simulink model "WorkshopB_1"  (R2016a)
settings: Solver=ode45  SolverMode=SingleTasking  StartTime=0.0  StopTime=5  RelTol=1e-3
values from neighbouring files (symbols this model uses):
  dm = dm*eps_dm    (= 1.3528e-05)    [param.m]
  Dpos = double(D)    [param.m]
  Fc = 0.0013    [param.m]
  Ipos = double(I)    [param.m]
  Jeq = eps_Jeq*Jeq    (= 2.20476e-05)    [param.m]
  Kemf = 1/(137*2*pi/60)    (= 0.0697028947848)    [param.m]
  Km = 69.7E-3    (= 0.0697)    [param.m]
  n = 1    [param.m]
  Npos = double(N)    [param.m]
  Ppos = double(P)    [param.m]
  R = s*s + s*N    [PID_calc.m]    (also in param.m = 112)
  Ts = 5e-3    (= 0.005)    [param.m]
undefined symbols (not defined in the file or in its folder): DiscIntNeverNeededParam, sigbuilder_block
settings Model: Creator=sofianh  LastModifiedBy=diegogm
settings DataIOCC: LimitDataPoints=on  SaveFormat=Array
settings OptimizationCC: BlockReduction=off  BooleanDataType=off
settings DebuggingCC: SaveWithParameterizedLinksMsg=none  UnderspecifiedInitializationDetection=Classic  MergeDetectMultiDrivingBlocksExec=none  SignalResolutionControl=TryResolveAllWithWarning
settings HardwareCC: ProdBitPerPointer=32  ProdLargestAtomicFloat=None  ProdIntDivRoundTo=Undefined  ProdEndianess=Unspecified  ProdWordSize=32  ProdHWDeviceType=32-bit Generic  TargetUnknown=on
settings ModelReferenceCC: PropagateSignalLabelsOutOfModel=off
settings ConfigComp: CovModelRefEnable=Off  CovSFcnEnable=off

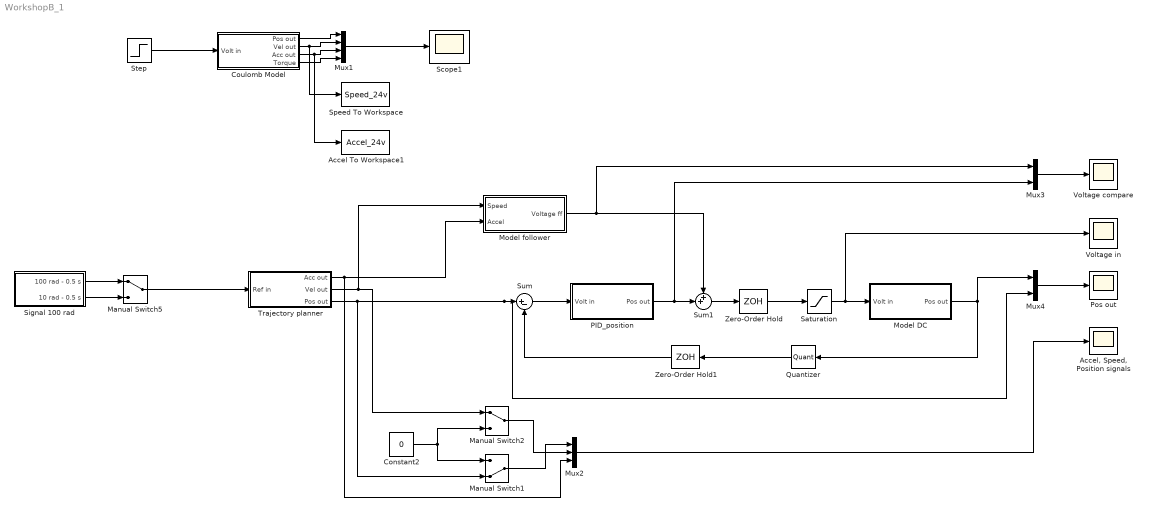
== system WorkshopB_1 ==
  Accel To Workspace1 : ToWorkspace  VariableName=Accel_24v  SaveFormat=Timeseries  SampleTime=-1
  "Accel, Speed, Position signals" : Scope
  Constant2 : Constant  Value=0
  Coulomb Model : Subsystem
  Manual Switch1 : ManualSwitch  CurrentSetting=0
  Manual Switch2 : ManualSwitch
  Manual Switch5 : ManualSwitch
  "Model DC " : Subsystem
  Model follower : Subsystem
  Mux1 : Mux
  Mux2 : Mux  Inputs=3
  Mux3 : Mux  Inputs=2
  Mux4 : Mux  Inputs=2
  PID_position : Subsystem
  Pos out : Scope
  Quantizer : Quantizer  QuantizationInterval=Pulses  SampleTime=Ts
  Saturation : Saturate  UpperLimit=24  LowerLimit=-24
  Scope1 : Scope
  Signal 100 rad : Subsystem  Tag=STV Subsys  LoadFcn=sigbuilder_block('load',[437.6 199.2 550.4 400 ]);  StartFcn=sigbuilder_block('start');  StopFcn=sigbuilder_block('stop');  ClipboardFcn=sigbuilder_block('clipboard');  mask(Sigbuilder block){}
      mask help: Simulink:masks:SigbuilderBlock_MD
      mask init:
      | if ~strcmp(get_param(bdroot(gcbh),'SimulationStatus'),'stopped') tuvar = sigbuilder_block('maskInit'); end
      settings: CopyFcn=sigbuilder_block('copy');  DeleteFcn=sigbuilder_block('delete');  ModelCloseFcn=sigbuilder_block('modelClose');  PreSaveFcn=sigbuilder_block('preSave');  PauseFcn=sigbuilder_block('pause');  ContinueFcn=sigbuilder_block('continue');  NameChangeFcn=sigbuilder_block('namechange');  OpenFcn=sigbuilder_block('open',[437.6 199.2 550.4 400 ]);  CloseFcn=sigbuilder_block('close');
      mask Display: plot(0, 0, 100, 100,[2, 2, 32, 32, 2], [68, 8, 8, 68, 68],[32, 2], [38, 38], [32, 19, 2],[53, 60, 44], [32, 17, 17, 2],[16, 16, 31, 31]);txt = getActiveGroup(gcbh);text(2, 100, txt,'verticalAlignment', 'top');
  Speed To Workspace : ToWorkspace  VariableName=Speed_24v  SaveFormat=Timeseries  SampleTime=-1
  Step : Step  Time=0  After=24  SampleTime=0
  Sum : Sum  Inputs=|+-
  Sum1 : Sum  Inputs=++|
  Trajectory planner : Subsystem
  Voltage compare : Scope
  Voltage in : Scope
  Zero-Order Hold : ZeroOrderHold  SampleTime=Ts
  Zero-Order Hold1 : ZeroOrderHold  SampleTime=Ts
  wires:
  Mux1/1 -> Scope1/1
  Coulomb Model/1(Pos out) -> Mux1/1
  Step/1 -> Coulomb Model/1(Volt in)
  Coulomb Model/2(Vel out) -> Speed To Workspace/1, Mux1/2
  Coulomb Model/3(Acc out) -> Accel To Workspace1/1, Mux1/3
  Coulomb Model/4(Torque) -> Mux1/4
  Mux2/1 -> "Accel, Speed, Position signals"/1
  Manual Switch1/1 -> Mux2/1
  Manual Switch2/1 -> Mux2/2
  Constant2/1 -> Manual Switch2/2, Manual Switch1/1
  Sum/1 -> PID_position/1(Volt in)
  "Model DC "/1(Pos out) -> Quantizer/1, Mux4/1
  PID_position/1(Pos out) -> Mux3/2, Sum1/2
  Mux3/1 -> Voltage compare/1
  Model follower/1(Voltage ff) -> Sum1/1, Mux3/1
  Mux4/1 -> Pos out/1
  Trajectory planner/1("Acc out ") -> Model follower/2(Accel), Mux2/3
  Trajectory planner/2(Vel out) -> Manual Switch2/1, Model follower/1(Speed)
  Trajectory planner/3("Pos out ") -> Mux4/2, Sum/1, Manual Switch1/2
  Sum1/1 -> Zero-Order Hold/1
  Quantizer/1 -> Zero-Order Hold1/1
  Zero-Order Hold1/1 -> Sum/2
  Manual Switch5/1 -> Trajectory planner/1(Ref in)
  Signal 100 rad/1(100 rad - 0.5 s) -> Manual Switch5/1
  Signal 100 rad/2(10 rad - 0.5 s) -> Manual Switch5/2
  Zero-Order Hold/1 -> Saturation/1
  Saturation/1 -> Voltage in/1, "Model DC "/1("Volt in ")

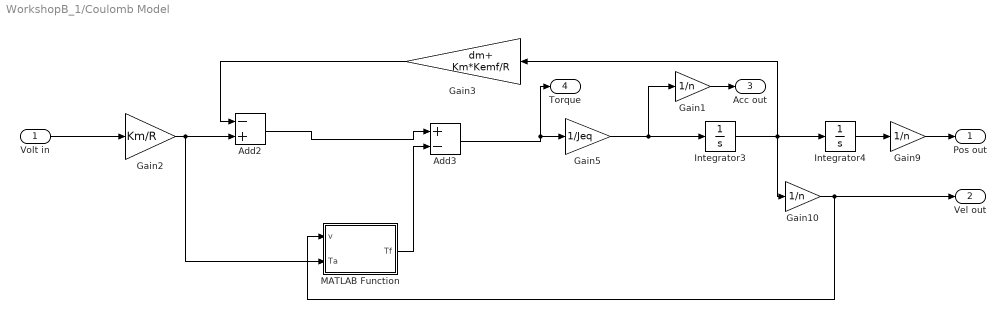
== system WorkshopB_1/Coulomb Model ==
  Volt in : Inport
  Add2 : Sum  Inputs=-+
  Add3 : Sum  Inputs=+-
  Gain1 : Gain  Gain=1/n
  Gain10 : Gain  Gain=1/n
  Gain2 : Gain  Gain=Km/R
  Gain3 : Gain  Gain=dm+ Km*Kemf/R
  Gain5 : Gain  Gain=1/Jeq
  Gain9 : Gain  Gain=1/n
  Integrator3 : Integrator
  Integrator4 : Integrator
  MATLAB Function : MATLAB Function  TreatAsAtomicUnit=on
  Pos out : Outport
  Vel out : Outport  Port=2
  Acc out : Outport  Port=3
  Torque : Outport  Port=4
  wires:
  Gain2/1 -> MATLAB Function/2(Ta), Add2/2
  Integrator3/1 -> Integrator4/1, Gain10/1, Gain3/1
  Gain3/1 -> Add2/1
  Gain5/1 -> Integrator3/1, Gain1/1
  Integrator4/1 -> Gain9/1
  Gain10/1 -> Vel out/1, MATLAB Function/1(v)
  Volt in/1 -> Gain2/1
  Add3/1 -> Torque/1, Gain5/1
  Add2/1 -> Add3/1
  MATLAB Function/1(Tf) -> Add3/2
  Gain9/1 -> Pos out/1
  Gain1/1 -> Acc out/1

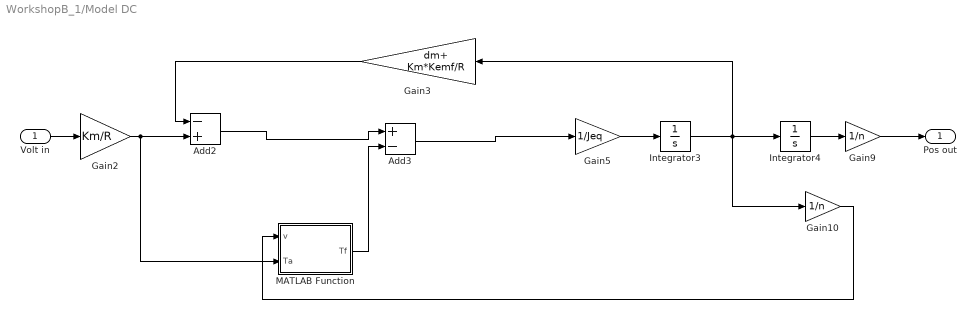
== system WorkshopB_1/Model DC  ==
  "Volt in " : Inport
  Add2 : Sum  Inputs=-+
  Add3 : Sum  Inputs=+-
  Gain10 : Gain  Gain=1/n
  Gain2 : Gain  Gain=Km/R
  Gain3 : Gain  Gain=dm+ Km*Kemf/R
  Gain5 : Gain  Gain=1/Jeq
  Gain9 : Gain  Gain=1/n
  Integrator3 : Integrator
  Integrator4 : Integrator
  MATLAB Function : MATLAB Function  TreatAsAtomicUnit=on
  Pos out : Outport
  wires:
  Gain2/1 -> MATLAB Function/2(Ta), Add2/2
  Integrator3/1 -> Integrator4/1, Gain10/1, Gain3/1
  Gain3/1 -> Add2/1
  Gain5/1 -> Integrator3/1
  Integrator4/1 -> Gain9/1
  Gain10/1 -> MATLAB Function/1(v)
  Add3/1 -> Gain5/1
  Add2/1 -> Add3/1
  MATLAB Function/1(Tf) -> Add3/2
  "Volt in "/1 -> Gain2/1
  Gain9/1 -> Pos out/1

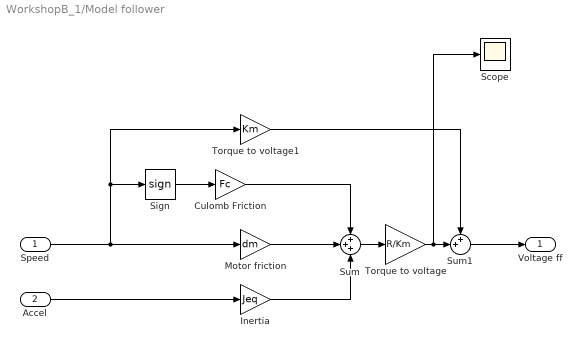
== system WorkshopB_1/Model follower ==
  Speed : Inport
  Accel : Inport  Port=2
  Culomb Friction : Gain  Gain=Fc
  "Inertia " : Gain  Gain=Jeq
  Motor friction : Gain  Gain=dm
  Scope : Scope
  Sign : Signum
  Sum : Sum  Inputs=+++
  Sum1 : Sum  Inputs=++|
  Torque to voltage : Gain  Gain=R/Km
  Torque to voltage1 : Gain  Gain=Km
  Voltage ff : Outport
  wires:
  Accel/1 -> "Inertia "/1
  Speed/1 -> Torque to voltage1/1, Sign/1, Motor friction/1
  "Inertia "/1 -> Sum/3
  Motor friction/1 -> Sum/2
  Sum/1 -> Torque to voltage/1
  Torque to voltage1/1 -> Sum1/1
  Torque to voltage/1 -> Scope/1, Sum1/2
  Sum1/1 -> Voltage ff/1
  Sign/1 -> Culomb Friction/1
  Culomb Friction/1 -> Sum/1

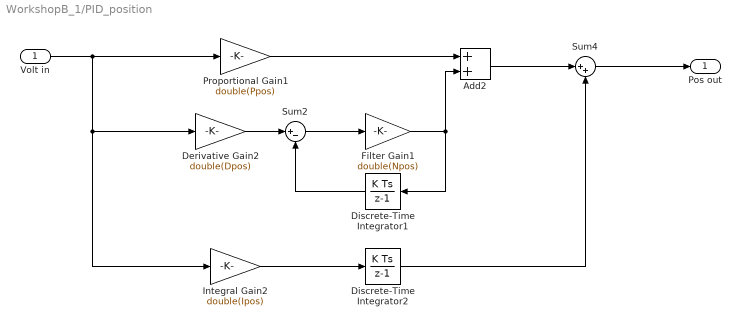
== system WorkshopB_1/PID_position ==
  Volt in : Inport
  Add2 : Sum
  Derivative Gain2 : Gain  Gain=double(Dpos)
  Discrete-Time Integrator1 : DiscreteIntegrator  InitialConditionSetting=State (most efficient)  SampleTime=Ts  ICPrevOutput=DiscIntNeverNeededParam  ICPrevScaledInput=DiscIntNeverNeededParam
  Discrete-Time Integrator2 : DiscreteIntegrator  InitialConditionSetting=State (most efficient)  SampleTime=Ts  ICPrevOutput=DiscIntNeverNeededParam  ICPrevScaledInput=DiscIntNeverNeededParam
  Filter Gain1 : Gain  Gain=double(Npos)
  Integral Gain2 : Gain  Gain=double(Ipos)
  Proportional Gain1 : Gain  Gain=double(Ppos)
  Sum2 : Sum  Inputs=|+-
  Sum4 : Sum  Inputs=|++
  Pos out : Outport
  wires:
  Discrete-Time Integrator2/1 -> Sum4/2
  Add2/1 -> Sum4/1
  Volt in/1 -> Integral Gain2/1, Derivative Gain2/1, Proportional Gain1/1
  Discrete-Time Integrator1/1 -> Sum2/2
  Sum2/1 -> Filter Gain1/1
  Derivative Gain2/1 -> Sum2/1
  Proportional Gain1/1 -> Add2/1
  Filter Gain1/1 -> Discrete-Time Integrator1/1, Add2/2
  Integral Gain2/1 -> Discrete-Time Integrator2/1
  Sum4/1 -> Pos out/1

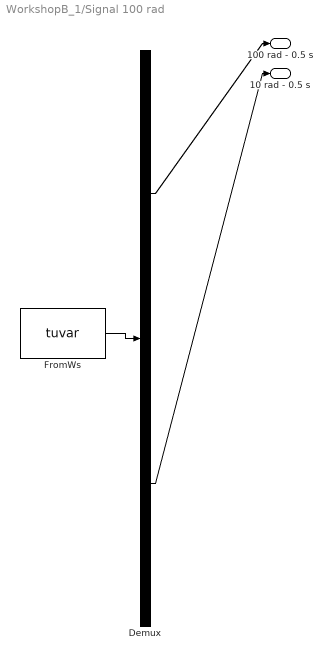
== system WorkshopB_1/Signal 100 rad ==
  Demux : Demux  Tag=STV Demux  Outputs=2
  FromWs : FromWorkspace  Tag=STV FromWs  VariableName=tuvar  SampleTime=0
      SigBuilderData=|
      | common.afterFinalStr = 'Extrapolate'
      | common.sampleTime = 0
      | dataSet.timeRange = [0 2]
      | dataSet.name = 'Group 1'
      | sbobj.Groups.Name = 'Group 1'
      | sbobj.Groups.Signals(1).Name = '100 rad - 0.5 s'
      | sbobj.Groups.Signals(1).XData = [0 0.5 0.5 1 1 1.5 1.5 2]
      | sbobj.Groups.Signals(1).YData = [200 200 0 0 -200 -200 0 0]
      | sbobj.Groups.Signals(2).Name = '10 rad - 0.5 s'
      | sbobj.Groups.Signals(2).XData = [0 0.5 0.5 1 1 1.5 1.5 2]
      | sbobj.Groups.Signals(2).YData = [20 20 0 0 -20 -20 0 0]
      | sbobj.Groups.TimeRange = [0 2]
  100 rad - 0.5 s : Outport  Tag=STV Outport
  10 rad - 0.5 s : Outport  Tag=STV Outport  Port=2
  wires:
  FromWs/1 -> Demux/1
  Demux/1 -> 100 rad - 0.5 s/1
  Demux/2 -> 10 rad - 0.5 s/1

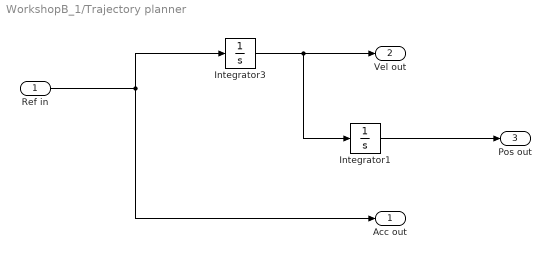
== system WorkshopB_1/Trajectory planner ==
  Ref in : Inport
  Integrator1 : Integrator
  Integrator3 : Integrator
  "Acc out " : Outport
  Vel out : Outport  Port=2
  "Pos out " : Outport  Port=3
  wires:
  Integrator3/1 -> Integrator1/1, Vel out/1
  Ref in/1 -> Integrator3/1, "Acc out "/1
  Integrator1/1 -> "Pos out "/1

== matlab function WorkshopB_1/Coulomb Model/MATLAB Function ==
  data: v input; Tf output; Ta input
function Tf = fcn(v,Ta)
Tc = 1e-3;
dv = 1e-1;
if abs(v) < dv
    if abs(Ta) > Tc
        Tf = Tc*sign(Ta);
    else
        Tf = Ta;
    end
else
    Tf = Tc*sign(v);
end

== matlab function WorkshopB_1/Model DC /MATLAB Function ==
  data: v input; Tf output; Ta input
function Tf = fcn(v,Ta)
Tc = 1e-3;
dv = 1e-1;
if abs(v) < dv
    if abs(Ta) > Tc
        Tf = Tc*sign(Ta);
    else
        Tf = Ta;
    end
else
    Tf = Tc*sign(v);
end
